simulink subsystem "MT"  (R2024a)
settings: Solver=VariableStepAuto  StartTime=0.0  StopTime=10.0  RelTol=1e-3
settings Model: Creator=nicol  LastModifiedBy=nicol

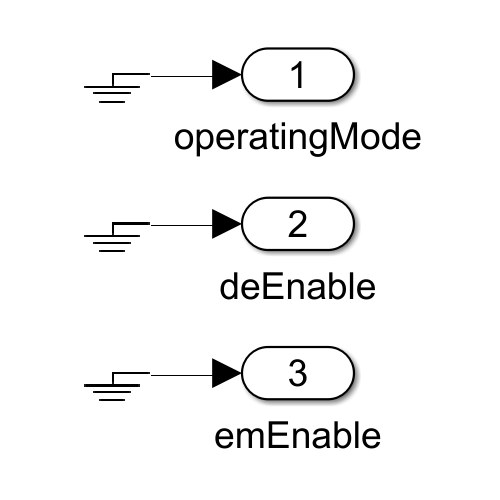
[thumbnail: Simulink's stored preview of the top-level diagram]
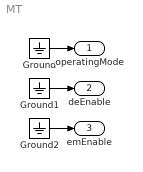
== system MT ==
  Ground : Ground
  Ground1 : Ground
  Ground2 : Ground
  operatingMode : Outport
  deEnable : Outport  Port=2
  emEnable : Outport  Port=3
  wires:
  Ground/1 -> operatingMode/1
  Ground1/1 -> deEnable/1
  Ground2/1 -> emEnable/1
